simulink model "WaterProp_R2015b"  (R2015b)
settings: Solver=FixedStepDiscrete  StartTime=0.0  StopTime=19.5  FixedStep=1  MaxStep=1  RelTol=1e-3
libraries: simulink x2
settings Model: Creator=awohlfei  LastModifiedBy=drhf
settings DataIOCC: SaveFormat=Array  SignalLoggingSaveFormat=ModelDataLogs  SaveTime=off
settings OptimizationCC: ExpressionDepthLimit=2147483647
settings DebuggingCC: UnderspecifiedInitializationDetection=Classic  MergeDetectMultiDrivingBlocksExec=none  SolverPrmCheckMsg=warning  FcnCallInpInsideContextMsg=EnableAllAsWarning  StateNameClashWarn=warning
settings HardwareCC: ProdBitPerPointer=32  ProdLargestAtomicFloat=None  ProdIntDivRoundTo=Undefined  ProdEndianess=Unspecified  ProdWordSize=32  ProdHWDeviceType=32-bit Generic
settings GRTTargetCC: GeneratePreprocessorConditionals=Disable all
settings ConfigComp: CovModelRefEnable=Off

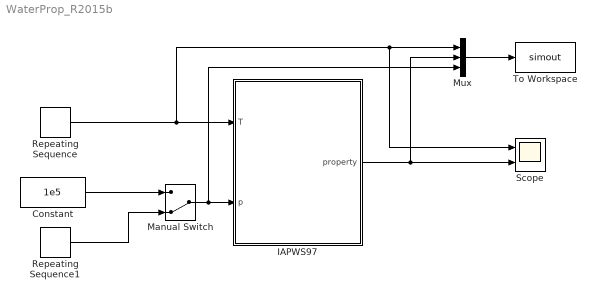
== system WaterProp_R2015b ==
  Constant : Constant  Value=1e5
  IAPWS97 : Subsystem  mask{PROPERTY=SATURATIONTEMPERATURE}
      mask TypeOptions PROPERTY: DENSITY | HEAT_CAPACITY | THERMAL_CONDUCTIVITY | VISCOSITY | ENTHALPY | ENTROPY | PRANDTL | SPECIFIC_VOLUME | EVAPORATION_ENTHALPY | VAPOURPRESSURE | SATURATIONTEMPERATURE | SATURATIONPROPERTY | TEMPERATURE_CONDUCTIVITY | ENTHALPY2TEMPERATURE
  Manual Switch : ManualSwitch  CurrentSetting=0
  Mux : Mux  Inputs=3
  Repeating Sequence : simulink/Sources/Repeating Sequence  rep_seq_t=[0 19 21]  rep_seq_y=[10 200 200]
  Repeating Sequence1 : simulink/Sources/Repeating Sequence  rep_seq_t=[0 19 21]  rep_seq_y=[600 3e5 3e5]
  Scope : Scope  NumInputPorts=2
  To Workspace : ToWorkspace  VariableName=simout  SampleTime=1
  wires:
  Repeating Sequence/1 -> Scope/1, Mux/1, IAPWS97/1(T)
  IAPWS97/1(property) -> Scope/2, Mux/2
  Mux/1 -> To Workspace/1
  Constant/1 -> Manual Switch/1
  Repeating Sequence1/1 -> Manual Switch/2
  Manual Switch/1 -> Mux/3, IAPWS97/2(p)

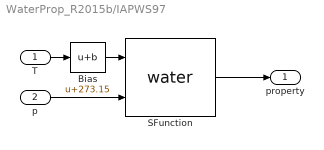
== system WaterProp_R2015b/IAPWS97 ==
  T : Inport
  p : Inport  Port=2
  Bias : Bias  Bias=273.15
  SFunction : S-Function  FunctionName=water  Parameters=PROPERTY  SFunctionDeploymentMode=off  EnableBusSupport=off
  property : Outport
  wires:
  T/1 -> Bias/1
  p/1 -> SFunction/2
  SFunction/1 -> property/1
  Bias/1 -> SFunction/1
